simulink model "ART25_full_car_old"  (R2022a)
settings: Solver=FixedStepAuto  StartTime=0.0  StopTime=10  FixedStep=sim_TimeStep  RelTol=1e-3
undefined symbols (not defined in the file): param, vx0, yaw_rate0
settings Model: Creator=jutri  LastModifiedBy=Usuario
settings DataIOCC: SaveFormat=Array
settings ModelReferenceCC: EnableRefExpFcnMdlSchedulingChecks=off
settings RTWCC: Description=Generic Real-Time Target

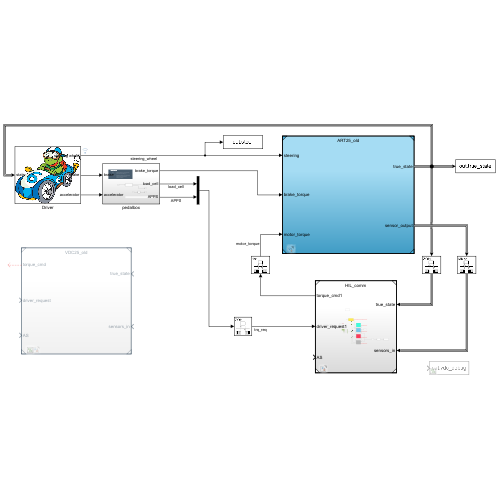
[thumbnail: Simulink's stored preview of the top-level diagram]
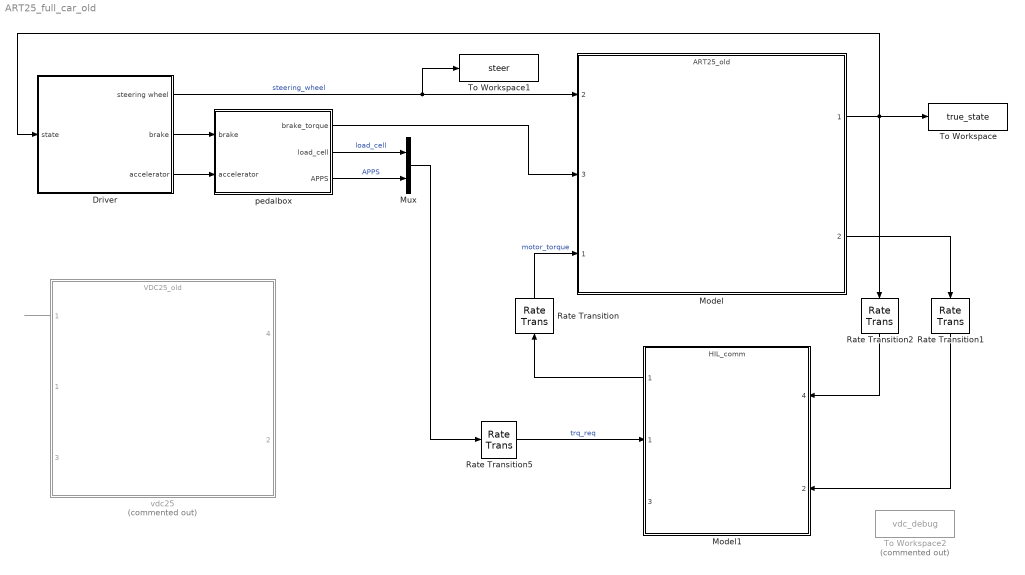
== system ART25_full_car_old ==
  Driver : Subsystem
      mask Display: image('Driver_logo.jpeg');
  Model : ModelReference  ModelNameDialog=ART25_old.slx  SimulationMode=Normal  ModelReferenceVersion=1.2
      settings: PortSchema="{\"entries\":[{\"content\":{\"sides\":[{\"content\":{\"connectorIds\":[\"In2\",\"In3\",\"In1\"]},\"type\":\"ConnectorPlacement.EquallySpacedRectSide\",\"uuid\":\"34e73162-f48c-446a-824e-17dcc9cc6514\"},{\"content\":{\"connectorIds\":[\"Out1\",\"Out2\"],\"side\":\"RIGHT\"},\"type\":\"ConnectorPlacement.EquallySpacedRectSide\",\"uuid\":\"74737ed4-0958-463a-8e43-c11e4d3189aa\"},{\"content\":{\"side\":\"TOP\"},\"type\":\"ConnectorPlacement.EquallySpacedRectSide\",\"uuid\":\"42fc3775-e72e-4fbb-8cdc-9d9cf3c0f815\"}]},\"type\":\"ConnectorPlacement.EquallySpacedConnector\",\"uuid\":\"6e643428-a593-4a05-90a3-6bfae895b914\"}],\"packageUris\":[\"http://schema.mathworks.com/mf0/Connector/R2020b\"],\"version\":\"1.0\"}"
  Model1 : ModelReference  ModelNameDialog=HIL_comm.slx  SimulationMode=Normal  ModelReferenceVersion=1.64
      settings: PortSchema="{\"entries\":[{\"content\":{\"sides\":[{\"content\":{\"connectorIds\":[\"Out1\",\"In1\",\"In3\"]},\"type\":\"ConnectorPlacement.EquallySpacedRectSide\",\"uuid\":\"04602d22-b9d7-40f7-b052-73f4143762fc\"},{\"content\":{\"connectorIds\":[\"In4\",\"In2\"],\"side\":\"RIGHT\"},\"type\":\"ConnectorPlacement.EquallySpacedRectSide\",\"uuid\":\"c5daacf6-0ad1-4531-a33a-b3ee5e66ed07\"},{\"content\":{\"connectorIds\":[],\"side\":\"TOP\"},\"type\":\"ConnectorPlacement.EquallySpacedRectSide\",\"uuid\":\"aa04230c-105f-45b7-b831-453931269445\"}]},\"type\":\"ConnectorPlacement.EquallySpacedConnector\",\"uuid\":\"55928aa8-a510-4f66-80b8-414931ecc3aa\"}],\"packageUris\":[\"http://schema.mathworks.com/mf0/Connector/R2020b\"],\"version\":\"1.0\"}"
  Mux : Mux  Inputs=2
  Rate Transition : RateTransition
  Rate Transition1 : RateTransition  Deterministic=off  OutPortSampleTime=vdc_TimeStep
  Rate Transition2 : RateTransition  OutPortSampleTime=vdc_TimeStep
  Rate Transition5 : RateTransition  OutPortSampleTime=vdc_TimeStep
  To Workspace : ToWorkspace  VariableName=true_state  SaveFormat=Structure With Time  SampleTime=-1
  To Workspace1 : ToWorkspace  VariableName=steer  SaveFormat=Structure  SampleTime=-1
  To Workspace2 : ToWorkspace  Commented=on  VariableName=vdc_debug  SaveFormat=Structure With Time  SampleTime=-1
  pedalbox : Subsystem
  vdc25 : ModelReference  Commented=on  ModelNameDialog=VDC25_old.slx  SimulationMode=Normal  ModelReferenceVersion=1.1
      settings: PortSchema="{\"entries\":[{\"content\":{\"sides\":[{\"content\":{\"connectorIds\":[\"Out1\",\"In1\",\"In3\"]},\"type\":\"ConnectorPlacement.EquallySpacedRectSide\",\"uuid\":\"da147370-b91a-4bb5-9c6b-40685e9dd617\"},{\"content\":{\"connectorIds\":[\"In4\",\"In2\"],\"side\":\"RIGHT\"},\"type\":\"ConnectorPlacement.EquallySpacedRectSide\",\"uuid\":\"d61eec38-a682-4bd1-95e6-e7fb713ea16a\"},{\"content\":{\"side\":\"TOP\"},\"type\":\"ConnectorPlacement.EquallySpacedRectSide\",\"uuid\":\"c636197e-c055-4dae-9ca6-30a202bee6bf\"}]},\"type\":\"ConnectorPlacement.EquallySpacedConnector\",\"uuid\":\"636ba342-8237-45ef-8445-7b2704fdba3c\"}],\"packageUris\":[\"http://schema.mathworks.com/mf0/Connector/R2020b\"],\"version\":\"1.0\"}"
  wires:
  Driver/1(steering wheel) -> To Workspace1/1, Model/2  "steering_wheel"
  Model/2 -> Rate Transition1/1
  Driver/2(brake) -> pedalbox/1(brake)
  vdc25/1 -> ?
  Model/1 -> Driver/1(state), Rate Transition2/1, To Workspace/1
  Driver/3(accelerator) -> pedalbox/2(accelerator)
  pedalbox/1(brake_torque) -> Model/3
  pedalbox/2(load_cell) -> Mux/1  "load_cell"
  pedalbox/3(APPS) -> Mux/2  "APPS"
  Mux/1 -> Rate Transition5/1
  Rate Transition5/1 -> Model1/1  "trq_req"
  Rate Transition1/1 -> Model1/2
  Rate Transition/1 -> Model/1  "motor_torque"
  Rate Transition2/1 -> Model1/4
  Model1/1 -> Rate Transition/1

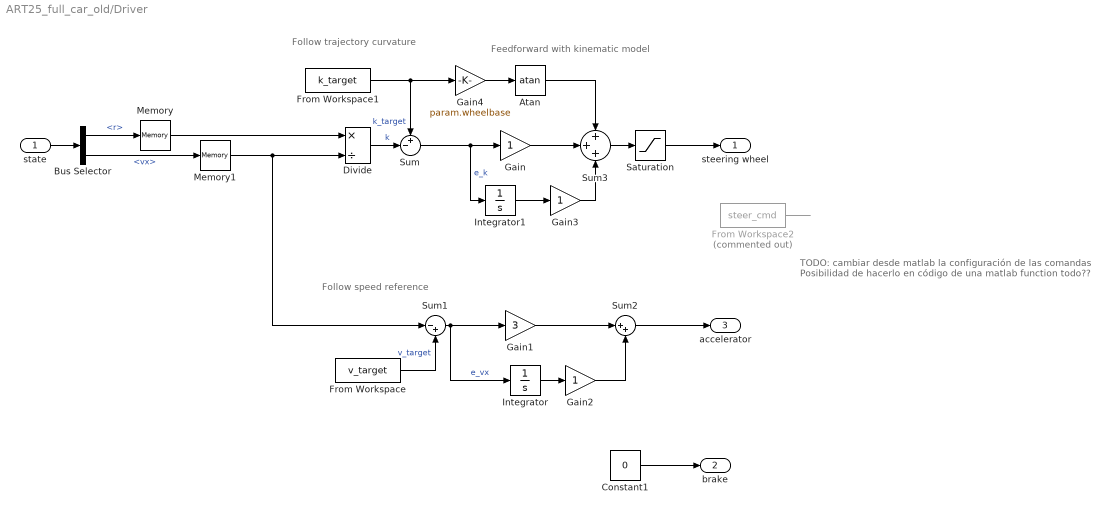
== system ART25_full_car_old/Driver ==
  note: TODO: cambiar desde matlab la configuración de las comandas
      | Posibilidad de hacerlo en código de una matlab function todo??
  note: Feedforward with kinematic model
  note: Follow trajectory curvature
  note: Follow speed reference
  state : Inport
  Atan : Trigonometry  Operator=atan
  Bus Selector : BusSelector  OutputSignals=r,vx
  Constant1 : Constant  Value=0
  Divide : Product  Inputs=*/
  From Workspace : FromWorkspace  VariableName=v_target
  From Workspace1 : FromWorkspace  VariableName=k_target
  From Workspace2 : FromWorkspace  Commented=on  VariableName=steer_cmd
  Gain : Gain
  Gain1 : Gain  Gain=3
  Gain2 : Gain
  Gain3 : Gain
  Gain4 : Gain  Gain=param.wheelbase
  Integrator : Integrator
  Integrator1 : Integrator
  Memory : Memory  InitialCondition=yaw_rate0
  Memory1 : Memory  InitialCondition=vx0
  Saturation : Saturate  UpperLimit=0.3  LowerLimit=-0.3
  Sum : Sum  Inputs=+-|
  Sum1 : Sum  Inputs=|-+
  Sum2 : Sum  Inputs=|++
  Sum3 : Sum  Inputs=+++
  steering wheel : Outport
  brake : Outport  Port=2
  accelerator : Outport  Port=3
  wires:
  Gain1/1 -> Sum2/1
  Constant1/1 -> brake/1
  state/1 -> Bus Selector/1
  Bus Selector/1 -> Memory/1  "<r>"
  Bus Selector/2 -> Memory1/1  "<vx>"
  Divide/1 -> Sum/2  "k"
  Sum1/1 -> Integrator/1, Gain1/1  "e_vx"
  From Workspace1/1 -> Gain4/1, Sum/1  "k_target"
  Sum2/1 -> accelerator/1
  Integrator/1 -> Gain2/1
  Gain2/1 -> Sum2/2
  Integrator1/1 -> Gain3/1
  Sum/1 -> Integrator1/1, Gain/1  "e_k"
  Sum3/1 -> Saturation/1
  Gain3/1 -> Sum3/3
  Gain/1 -> Sum3/2
  Saturation/1 -> steering wheel/1
  From Workspace/1 -> Sum1/2  "v_target"
  Gain4/1 -> Atan/1
  Atan/1 -> Sum3/1
  Memory/1 -> Divide/1
  Memory1/1 -> Divide/2, Sum1/1
  From Workspace2/1 -> ?

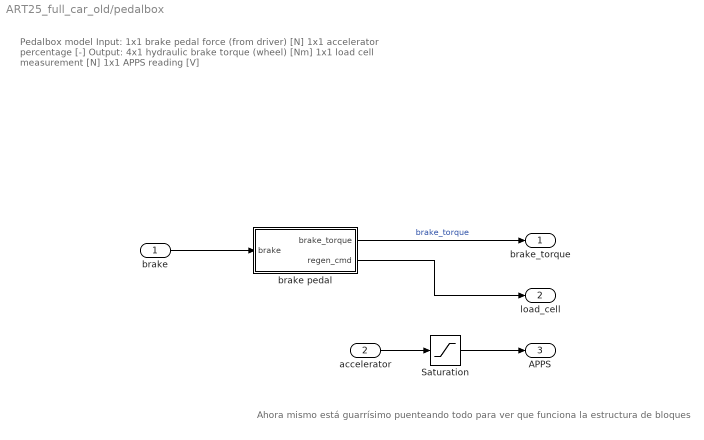
== system ART25_full_car_old/pedalbox ==
  note: Ahora mismo está guarrísimo puenteando todo para ver que funciona la estructura de bloques
  note: Pedalbox model
      |
      | Input: 1x1 brake pedal force (from driver) [N]
      | 1x1 accelerator percentage [-]
      |
      | Output: 4x1 hydraulic brake torque (wheel) [Nm]
      | 1x1 load cell measurement [N]
      | 1x1 APPS reading [V]
  brake : Inport
  accelerator : Inport  Port=2
  Saturation : Saturate  UpperLimit=1  LowerLimit=-1
  brake pedal : Subsystem
  brake_torque : Outport
  load_cell : Outport  Port=2
  APPS : Outport  Port=3
  wires:
  brake pedal/1(brake_torque) -> brake_torque/1  "brake_torque"
  brake pedal/2(regen_cmd) -> load_cell/1
  brake/1 -> brake pedal/1(brake)
  accelerator/1 -> Saturation/1
  Saturation/1 -> APPS/1

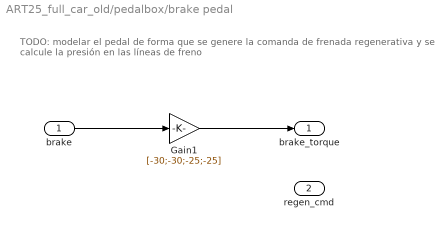
== system ART25_full_car_old/pedalbox/brake pedal ==
  note: TODO: modelar el pedal de forma que se genere la comanda de frenada regenerativa y se calcule la presión en las líneas de freno
  brake : Inport
  Gain1 : Gain  Gain=[-30;-30;-25;-25]
  brake_torque : Outport
  regen_cmd : Outport  Port=2
  wires:
  Gain1/1 -> brake_torque/1
  brake/1 -> Gain1/1
